simulink model "sobelFilter2024ab"  (R2024a)
settings: Solver=FixedStepDiscrete  StartTime=0.0  StopTime=2  RelTol=1e-3
values from neighbouring files (symbols this model uses):
  coefficients = [1 0 -1 ... (first row only)    [setup.m]
  R = 752    [setup.m]
undefined symbols (not defined in the file or in its folder): gray
libraries: hdlsllib x9, visionhdlio x4, visionsources x1
Description:
  | Sobel Edge Detection Using the MATLAB(R) Function Block
  | This example shows how to use HDL Coder(TM) to check,
  | generate, and verify HDL code for a Sobel Edge Detection
  | block built using the MATLAB Function block.
settings Model: FPTRunName=Active  Creator=The MathWorks, Inc.  LastModifiedBy=obb2733
settings SolverCC: AlgebraicLoopSolver=TrustRegion
settings DataIOCC: LimitDataPoints=on  SaveFormat=Array  SignalLogging=off  ReturnWorkspaceOutputs=off
settings OptimizationCC: BlockReduction=off  ConditionallyExecuteInputs=off  DefaultParameterBehavior=Inlined  ExpressionDepthLimit=2147483647  InitFltsAndDblsToZero=on  EfficientMapNaN2IntZero=off  LifeSpan=inf
settings DebuggingCC: AlgebraicLoopMsg=error  SaveWithParameterizedLinksMsg=none  UnderspecifiedInitializationDetection=Classic  MergeDetectMultiDrivingBlocksExec=none  SignalResolutionControl=TryResolveAllWithWarning  MultiTaskDSMMsg=warning  MultiTaskCondExecSysMsg=none  SingleTaskRateTransMsg=error  IntegerOverflowMsg=none  ParameterPrecisionLossMsg=none  FcnCallInpInsideContextMsg=warning  UnconnectedInputMsg=warning  UnconnectedOutputMsg=warning  UnconnectedLineMsg=warning  AllowSymbolicDim=off  StateNameClashWarn=warning  StrictBusMsg=ErrorOnBusTreatedAsVector  SFUnexpectedBacktrackingDiag=warning  SFNoUnconditionalDefaultTransitionDiag=warning  SFExecutionAtInitializationDiag=none  IntegerSaturationMsg=none  ArithmeticOperatorsInVariantConditions=warning
settings HardwareCC: ProdBitPerPointer=32  ProdBitPerSizeT=32  ProdBitPerPtrDiffT=32  ProdLargestAtomicFloat=None  ProdIntDivRoundTo=Undefined  ProdEndianess=Unspecified  ProdWordSize=32  ProdHWDeviceType=ASIC/FPGA  TargetHWDeviceType=32-bit Generic  ProdEqTarget=off
settings ModelReferenceCC: EnableRefExpFcnMdlSchedulingChecks=on  PropagateSignalLabelsOutOfModel=off
settings SFSimCC: SimUseLocalCustomCode=off  CustomCodeUndefinedFunction=UseInterfaceOnly
settings RTWCC: RTWUseLocalCustomCode=off  GPUComputeCapability=3.5  DLArmComputeVersion=19.05
settings CodeAppCC: StateflowObjectComments=on
settings GRTTargetCC: TargetFcnLib=ansi_tfl_tmw.mat  TargetLangStandard=C89/C90 (ANSI)  CombineOutputUpdateFcns=off  GRTInterface=on
settings ConfigComp: CovMetricSettings=dw  CovSaveCumulativeToWorkspaceVar=on  CovSaveSingleToWorkspaceVar=on  CovExternalEMLEnable=off

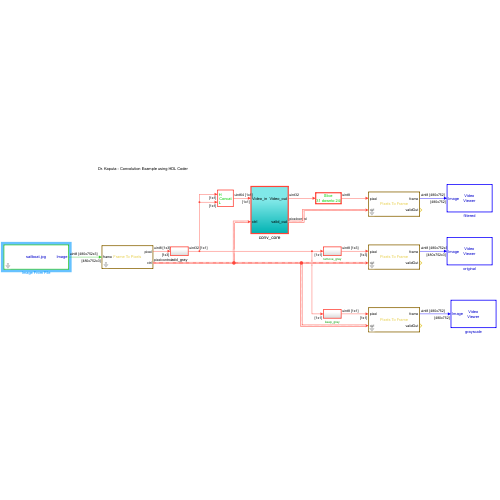
[thumbnail: Simulink's stored preview of the top-level diagram]
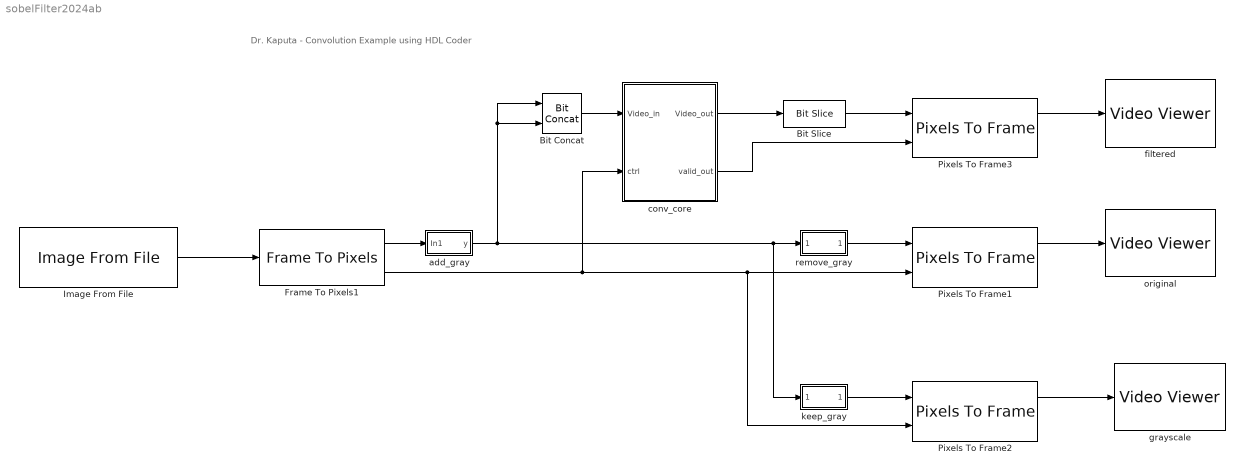
== system sobelFilter2024ab ==
  note: Dr. Kaputa - Convolution Example using HDL Coder
  Bit Concat : hdlsllib/Logic and Bit Operations/Bit Concat  numInputs=2
  Bit Slice : hdlsllib/Logic and Bit Operations/Bit Slice  lidx=31  ridx=24
  Frame To Pixels1 : visionhdlio/Frame To Pixels  NumComponents=3  NumPixels=1  VideoFormat=Custom  ActivePixelsPerLine=R  ActiveVideoLines=C  TotalPixelsPerLine=R  TotalVideoLines=C  StartingActiveLine=1  FrontPorch=0  SampleTime=0  VideoFormatCache=Custom  ActivePixelsPerLineCache=R  ActiveVideoLinesCache=C  TotalPixelsPerLineCache=R  TotalVideoLinesCache=C  StartingActiveLineCache=1  FrontPorchCache=0
  Image From File : visionsources/Image From File  Tag=vipblks_nd  FileName=sailboat.jpg  Ts=1  imagePorts=One multidimensional signal  OutPortLabels=R|G|B  ImageDataType=Inherit from input image  sdImageDataType=uint(8)  Signed=on  WordLength=16  FractionLengthMode=User-defined  FractionLength=15
  Pixels To Frame1 : visionhdlio/Pixels To Frame  NumComponents=3  NumPixels=1  VideoFormat=Custom  ActivePixelsPerLine=R  ActiveVideoLines=C  TotalPixelsPerLine=R  TotalVideoLines=C  VideoFormatCache=Custom  ActivePixelsPerLineCache=R  ActiveVideoLinesCache=C  TotalPixelsPerLineCache=R  TotalVideoLinesCache=C
  Pixels To Frame2 : visionhdlio/Pixels To Frame  NumComponents=1  NumPixels=1  VideoFormat=Custom  ActivePixelsPerLine=R  ActiveVideoLines=C  TotalPixelsPerLine=R  TotalVideoLines=C  VideoFormatCache=Custom  ActivePixelsPerLineCache=R  ActiveVideoLinesCache=C  TotalPixelsPerLineCache=R  TotalVideoLinesCache=C
  Pixels To Frame3 : visionhdlio/Pixels To Frame  NumComponents=1  NumPixels=1  VideoFormat=Custom  ActivePixelsPerLine=R  ActiveVideoLines=C  TotalPixelsPerLine=R  TotalVideoLines=C  VideoFormatCache=Custom  ActivePixelsPerLineCache=R  ActiveVideoLinesCache=C  TotalPixelsPerLineCache=R  TotalVideoLinesCache=C
  add_gray : Subsystem
  conv_core : Subsystem  TreatAsAtomicUnit=on
  filtered : VideoViewer  colormapValue=gray(256)  FigPos=[1 718 1280 622.666666666667]
  grayscale : VideoViewer  FigPos=[91 619.333333333333 1097.33333333333 520]
  keep_gray : Subsystem
  original : VideoViewer  FigPos=[1 725.333333333333 1280 622.666666666667]
  remove_gray : Subsystem
  wires:
  Image From File/1 -> Frame To Pixels1/1
  Pixels To Frame1/1 -> original/1
  Frame To Pixels1/2 -> conv_core/2(ctrl), Pixels To Frame1/2, Pixels To Frame2/2
  remove_gray/1(RGBVector) -> Pixels To Frame1/1
  Frame To Pixels1/1 -> add_gray/1(In1)
  add_gray/1(y) -> Bit Concat/2, Bit Concat/1, keep_gray/1(RGB), remove_gray/1(RGB)
  Pixels To Frame2/1 -> grayscale/1
  keep_gray/1(RGBVector) -> Pixels To Frame2/1
  Pixels To Frame3/1 -> filtered/1
  conv_core/1(Video_out) -> Bit Slice/1
  conv_core/2(valid_out) -> Pixels To Frame3/2
  Bit Concat/1 -> conv_core/1(Video_in)
  Bit Slice/1 -> Pixels To Frame3/1

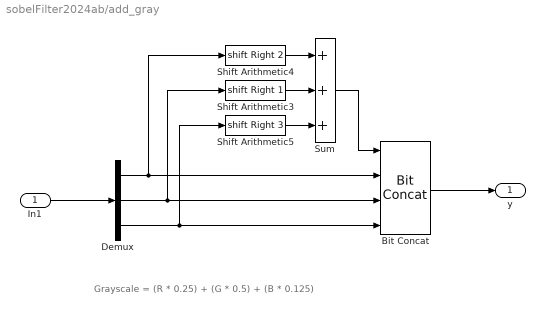
== system sobelFilter2024ab/add_gray ==
  note: Grayscale = (R * 0.25) + (G * 0.5) + (B * 0.125)
  In1 : Inport
  Bit Concat : hdlsllib/Logic and Bit Operations/Bit Concat  numInputs=4
  Demux : Demux  Outputs=3
  Shift Arithmetic3 : ArithShift  BitShiftNumber=1  BitShiftDirection=Right
  Shift Arithmetic4 : ArithShift  BitShiftNumber=2  BitShiftDirection=Right
  Shift Arithmetic5 : ArithShift  BitShiftNumber=3  BitShiftDirection=Right
  Sum : Sum  Inputs=+++  OutDataTypeStr=uint8
  y : Outport
  wires:
  Bit Concat/1 -> y/1
  In1/1 -> Demux/1
  Demux/2 -> Shift Arithmetic3/1, Bit Concat/3
  Demux/1 -> Shift Arithmetic4/1, Bit Concat/2
  Demux/3 -> Shift Arithmetic5/1, Bit Concat/4
  Sum/1 -> Bit Concat/1
  Shift Arithmetic4/1 -> Sum/1
  Shift Arithmetic3/1 -> Sum/2
  Shift Arithmetic5/1 -> Sum/3

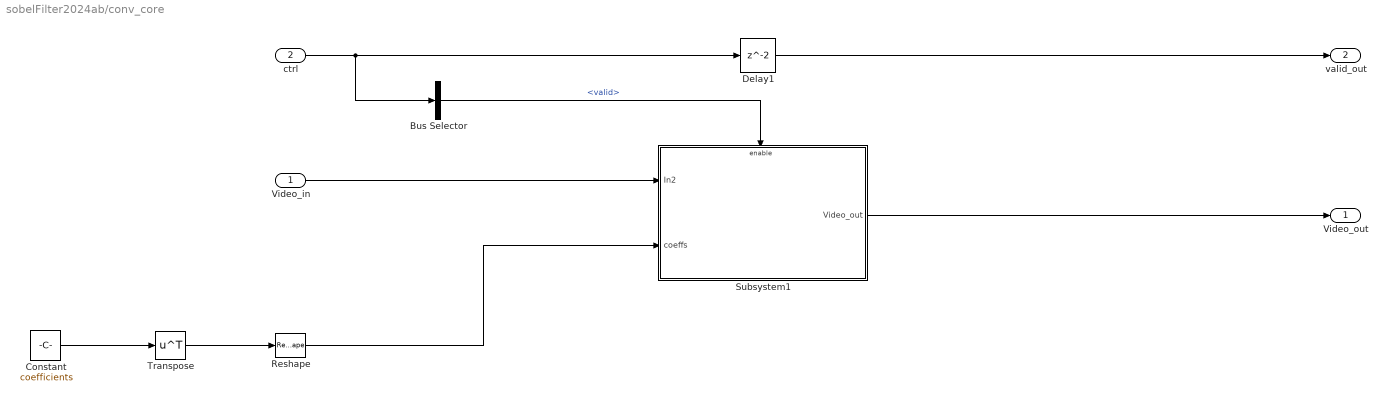
== system sobelFilter2024ab/conv_core ==
  Video_in : Inport
  ctrl : Inport  Port=2
  Bus Selector : BusSelector  OutputSignals=valid
  Constant : Constant  Value=coefficients  OutDataTypeStr=fixdt(1,16,12)  SampleTime=-1
  Delay1 : Delay  InitialCondition=0
  Reshape : Reshape
  Subsystem1 : Subsystem
  Transpose : Math  Operator=transpose
  Video_out : Outport  VectorParamsAs1DForOutWhenUnconnected=off
  valid_out : Outport  Port=2  VectorParamsAs1DForOutWhenUnconnected=off
  wires:
  Video_in/1 -> Subsystem1/1(In2)
  ctrl/1 -> Bus Selector/1, Delay1/1
  Bus Selector/1 -> Subsystem1/Enable  "<valid>"
  Subsystem1/1(Video_out) -> Video_out/1
  Reshape/1 -> Subsystem1/2(coeffs)
  Delay1/1 -> valid_out/1
  Constant/1 -> Transpose/1
  Transpose/1 -> Reshape/1

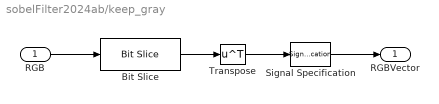
== system sobelFilter2024ab/keep_gray ==
  RGB : Inport
  Bit Slice : hdlsllib/Logic and Bit Operations/Bit Slice  lidx=31  ridx=24
  Signal Specification : SignalSpecification
  Transpose : Math  Operator=transpose  SignedPower=on
  RGBVector : Outport  VectorParamsAs1DForOutWhenUnconnected=off
  wires:
  RGB/1 -> Bit Slice/1
  Transpose/1 -> Signal Specification/1
  Signal Specification/1 -> RGBVector/1
  Bit Slice/1 -> Transpose/1

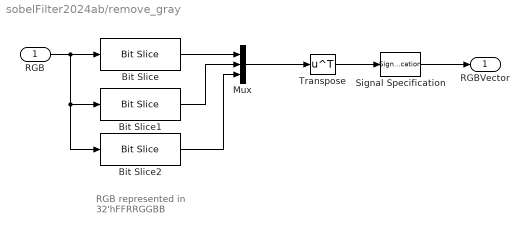
== system sobelFilter2024ab/remove_gray ==
  note: RGB represented in
      | 32'hFFRRGGBB
  RGB : Inport
  Bit Slice : hdlsllib/Logic and Bit Operations/Bit Slice  lidx=23  ridx=16
  Bit Slice1 : hdlsllib/Logic and Bit Operations/Bit Slice  lidx=15  ridx=8
  Bit Slice2 : hdlsllib/Logic and Bit Operations/Bit Slice  lidx=7  ridx=0
  Mux : Mux  Inputs=3
  Signal Specification : SignalSpecification
  Transpose : Math  Operator=transpose  SignedPower=on
  RGBVector : Outport  VectorParamsAs1DForOutWhenUnconnected=off
  wires:
  Signal Specification/1 -> RGBVector/1
  Transpose/1 -> Signal Specification/1
  RGB/1 -> Bit Slice/1, Bit Slice1/1, Bit Slice2/1
  Bit Slice1/1 -> Mux/2
  Bit Slice2/1 -> Mux/3
  Bit Slice/1 -> Mux/1
  Mux/1 -> Transpose/1

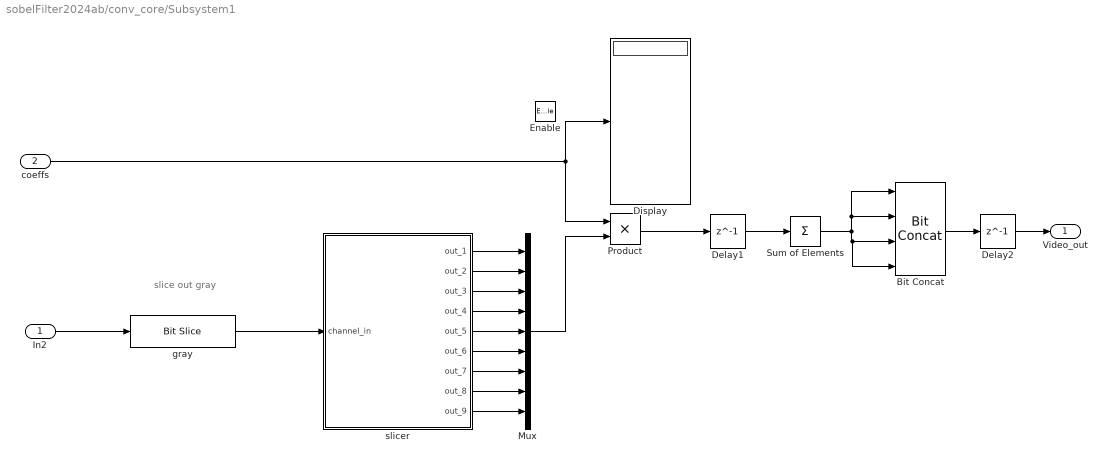
== system sobelFilter2024ab/conv_core/Subsystem1 ==
  note: slice out gray
  In2 : Inport
  coeffs : Inport  Port=2
  Enable : EnablePort
  Bit Concat : hdlsllib/Logic and Bit Operations/Bit Concat  numInputs=4
  Delay1 : Delay  DelayLength=1  InitialCondition=0
  Delay2 : Delay  DelayLength=1  InitialCondition=0
  Display : Display
      settings: Format=hex (Stored Integer)
  Mux : Mux  Inputs=9
  Product : Product  SaturateOnIntegerOverflow=on
  Sum of Elements : Sum  Inputs=+  OutDataTypeStr=uint8  SaturateOnIntegerOverflow=on
  gray : hdlsllib/Logic and Bit Operations/Bit Slice  lidx=31  ridx=24
  slicer : Subsystem
  Video_out : Outport  InitialOutput=[0]
  wires:
  slicer/1(out_1) -> Mux/1
  In2/1 -> gray/1
  slicer/9(out_9) -> Mux/9
  slicer/5(out_5) -> Mux/5
  slicer/7(out_7) -> Mux/7
  slicer/3(out_3) -> Mux/3
  slicer/6(out_6) -> Mux/6
  slicer/4(out_4) -> Mux/4
  slicer/2(out_2) -> Mux/2
  gray/1 -> slicer/1(channel_in)
  slicer/8(out_8) -> Mux/8
  Mux/1 -> Product/2
  coeffs/1 -> Product/1, Display/1
  Sum of Elements/1 -> Bit Concat/1, Bit Concat/2, Bit Concat/4, Bit Concat/3
  Product/1 -> Delay1/1
  Delay1/1 -> Sum of Elements/1
  Bit Concat/1 -> Delay2/1
  Delay2/1 -> Video_out/1

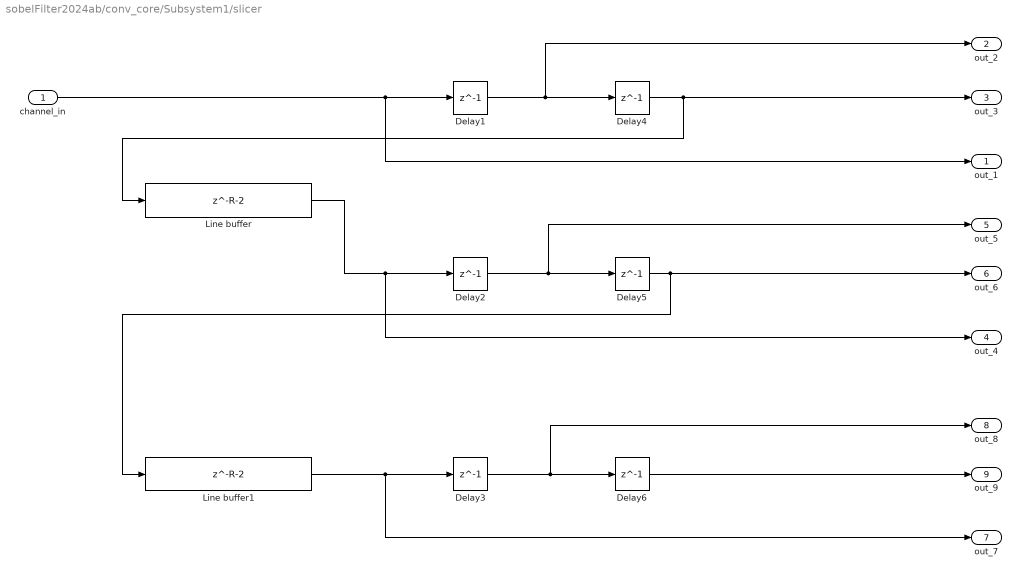
== system sobelFilter2024ab/conv_core/Subsystem1/slicer ==
  channel_in : Inport
  Delay{1..6} (6 alike) : Delay  DelayLength=1  InitialCondition=0
  Line buffer : Delay  DelayLength=R-2  InitialCondition=0
  Line buffer1 : Delay  DelayLength=R-2  InitialCondition=0
  out_1 : Outport  VectorParamsAs1DForOutWhenUnconnected=off
  out_2 : Outport  Port=2  VectorParamsAs1DForOutWhenUnconnected=off
  out_3 : Outport  Port=3  VectorParamsAs1DForOutWhenUnconnected=off
  out_4 : Outport  Port=4  VectorParamsAs1DForOutWhenUnconnected=off
  out_5 : Outport  Port=5  VectorParamsAs1DForOutWhenUnconnected=off
  out_6 : Outport  Port=6  VectorParamsAs1DForOutWhenUnconnected=off
  out_7 : Outport  Port=7  VectorParamsAs1DForOutWhenUnconnected=off
  out_8 : Outport  Port=8  VectorParamsAs1DForOutWhenUnconnected=off
  out_9 : Outport  Port=9  VectorParamsAs1DForOutWhenUnconnected=off
  wires:
  Delay4/1 -> Line buffer/1, out_3/1
  channel_in/1 -> out_1/1, Delay1/1
  Delay1/1 -> out_2/1, Delay4/1
  Delay3/1 -> out_8/1, Delay6/1
  Delay5/1 -> Line buffer1/1, out_6/1
  Delay6/1 -> out_9/1
  Line buffer/1 -> out_4/1, Delay2/1
  Line buffer1/1 -> out_7/1, Delay3/1
  Delay2/1 -> out_5/1, Delay5/1
